simulink model "PI_controller_antiwindup1b"  (R2019b)
settings: Solver=FixedStepAuto  StartTime=0.0  StopTime=6  FixedStep=0.005  RelTol=1e-3
settings Model: Creator=suvo  LastModifiedBy=suvo

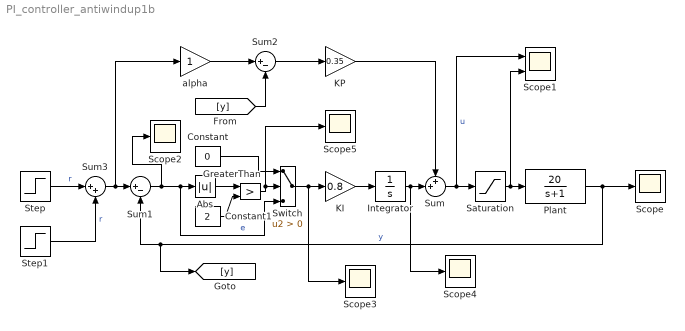
== system PI_controller_antiwindup1b ==
  Abs : Abs
  Constant : Constant  Value=0
  Constant1 : Constant  Value=2
  GreaterThan : RelationalOperator  Operator=>  OutDataTypeStr=boolean  RndMeth=Simplest
  Integrator : Integrator
  KI : Gain  Gain=0.8
  KP : Gain  Gain=0.35
  Plant : TransferFcn  Numerator=20  Denominator=[1 1]
  Saturation : Saturate  UpperLimit=0.05  LowerLimit=-0.05
  Scope{,2..5} (5 alike) : Scope
  Scope1 : Scope  NumInputPorts=2
  Step : Step  SampleTime=0
  Step1 : Step  Time=3  After=-1  SampleTime=0
  Sum : Sum  Inputs=++|
  Sum1 : Sum  Inputs=|+-
  Sum2 : Sum  Inputs=|+-
  Sum3 : Sum  Inputs=|++
  Switch : Switch  Criteria=u2 > Threshold
  alpha : Gain
  wires:
  KI/1 -> Integrator/1
  Plant/1 -> Scope/1, [y], Sum1/2  "y"
  Sum2/1 -> KP/1
  KP/1 -> Sum/1
  Integrator/1 -> Scope4/1, Sum/2
  Sum/1 -> Scope1/1, Saturation/1  "u"
  [y] -> Sum2/2
  alpha/1 -> Sum2/1
  Saturation/1 -> Scope1/2, Plant/1
  Step/1 -> Sum3/1  "r"
  Sum3/1 -> alpha/1, Sum1/1
  Step1/1 -> Sum3/2  "r"
  Constant/1 -> Switch/1
  Sum1/1 -> Scope2/1, Switch/3, Abs/1  "e"
  Switch/1 -> Scope3/1, KI/1
  Abs/1 -> GreaterThan/1
  Constant1/1 -> GreaterThan/2
  GreaterThan/1 -> Scope5/1, Switch/2
